simulink model "balancingController_QP_oneFoot"  (R2014b)
settings: Solver=FixedStepDiscrete  StartTime=0.0  StopTime=simulationTime  FixedStep=Ts  RelTol=1e-3
InitFcn:
  | initBalancingController_QP_oneFoot;
undefined symbols (not defined in the file): Aineq_F, amplitudesOscillationsOnOneFoot, bineq_F, directionOfOscillation, frequenciesOscillationsOnOneFoot, gainMomentum, gainsDCOM, gainsICOM, gainsPCOM, impedances, impedencesSat, increasingRatesImp, init_params_QP, localName, number_of_feet_on_ground, referenceParams, robotName, Ts
libraries: WBCLibrary x27
settings Model: Creator=daniele  LastModifiedBy=pucci
settings OptimizationCC: ExpressionDepthLimit=2147483647
settings DebuggingCC: UnderspecifiedInitializationDetection=Classic  MergeDetectMultiDrivingBlocksExec=none  FcnCallInpInsideContextMsg=EnableAllAsWarning  StateNameClashWarn=warning
settings SFSimCC: SimParseCustomCode=off
settings GRTTargetCC: CombineOutputUpdateFcns=off  GRTInterface=on

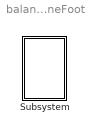
== system balancingController_QP_oneFoot ==
  Subsystem : Subsystem  mask{robotName=robotName, Ts=Ts, localName=localName}
      mask prompts: robotName "robot name"; localName "module name"

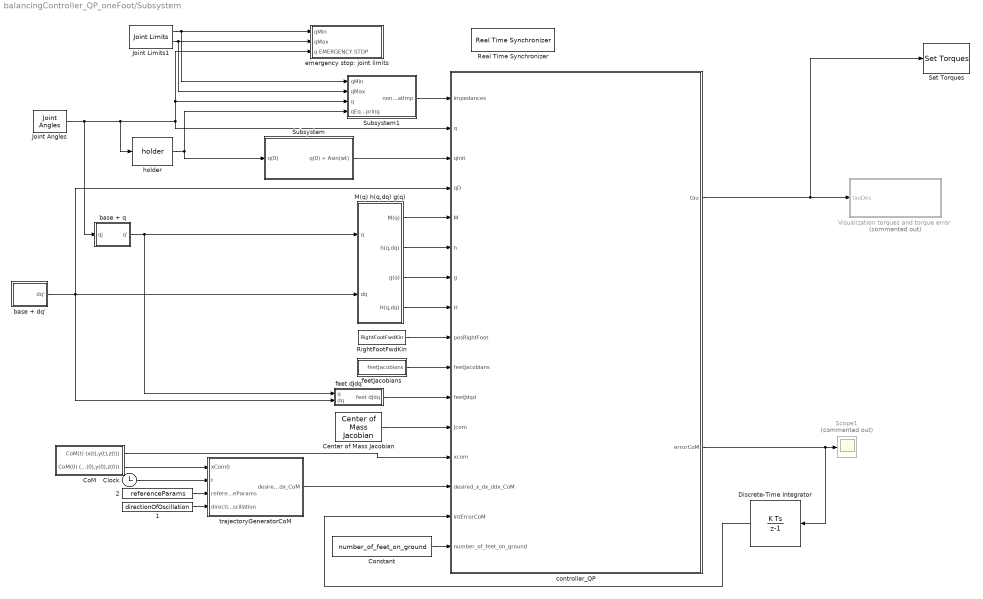
== system balancingController_QP_oneFoot/Subsystem ==
  " 1" : Constant  Value=directionOfOscillation
  " 2" : Constant  Value=referenceParams
  Center of Mass Jacobian : WBCLibrary/wholeBodyModel/Jacobians/Center of Mass Jacobian  robotName=robotName  localName=localName
  Clock : Clock
  "CoM " : Subsystem
  Constant : Constant  Value=number_of_feet_on_ground
  Discrete-Time Integrator : DiscreteIntegrator  InitialCondition=[0 0 0]  SampleTime=Ts
  Joint Angles : WBCLibrary/wholeBodyStates/Joint Angles  robotName=robotName  localName=localName
  Joint Limits1 : WBCLibrary/wholeBodyModel/Joint Limits  robotName=robotName  localName=localName
  M(q) h(q,dq) g(q) : Subsystem
  Real Time Synchronizer : WBCLibrary/Utilities/Real Time Synchronizer  Priority=-10  threadPeriod=Ts
  RightFootFwdKin : WBCLibrary/wholeBodyModel/Forward Kinematics/RightFootFwdKin  robotName=robotName  localName=localName
  Scope1 : Scope  Commented=on
      settings: SaveName=ScopeData6
  Set Torques : WBCLibrary/wholeBodyActuators/Set Torques  val=6  robotName=robotName  localName=localName
  Subsystem : Subsystem
  Subsystem1 : Subsystem
  Visualization torques and torque error : Subsystem  Commented=on
  base + dq' : Subsystem
  base + q : Subsystem
  controller_QP : Subsystem
  emergency stop: joint limits : Subsystem
  feet dJdq : Subsystem
  feetJacobians : Subsystem
  "holder " : WBCLibrary/Utilities/holder 
  trajectoryGeneratorCoM : MATLAB Function  TreatAsAtomicUnit=on
  wires:
  trajectoryGeneratorCoM/1(desired_x_dx_ddx_CoM) -> controller_QP/14(desired_x_dx_ddx_CoM)
  "CoM "/2(CoM(0) (x(0),y(0),z(0))) -> trajectoryGeneratorCoM/1(xCom0)
  RightFootFwdKin/1 -> controller_QP/9(posRightFoot)
  Discrete-Time Integrator/1 -> controller_QP/15(intErrorCoM)
  base + q/1(q') -> M(q) h(q,dq) g(q)/1(q), feet dJdq/1(q)
  M(q) h(q,dq) g(q)/3(g(q)) -> controller_QP/7(g)
  M(q) h(q,dq) g(q)/4(H(q,dq)) -> controller_QP/8(H)
  Center of Mass Jacobian/1 -> controller_QP/12(Jcom)
  feetJacobians/1(feetJacobians) -> controller_QP/10(feetJacobians)
  feet dJdq/1(feet dJdq) -> controller_QP/11(feetJdqd)
  "holder "/1 -> Subsystem1/4(qEquSpring), Subsystem/1(q(0))
  "CoM "/1(CoM(t) (x(t),y(t),z(t))) -> controller_QP/13(xcom)
  base + dq'/1(dq') -> controller_QP/4(qD), M(q) h(q,dq) g(q)/2(dq), feet dJdq/2(dq)
  M(q) h(q,dq) g(q)/1(M(q)) -> controller_QP/5(M)
  M(q) h(q,dq) g(q)/2(h(q,dq)) -> controller_QP/6(h)
  controller_QP/2(errorCoM) -> Scope1/1, Discrete-Time Integrator/1
  Constant/1 -> controller_QP/16(number_of_feet_on_ground)
  controller_QP/1(tau) -> Visualization torques and torque error/1(tauDes), Set Torques/1
  " 2"/1 -> trajectoryGeneratorCoM/3(referenceParams)
  Clock/1 -> trajectoryGeneratorCoM/2(t)
  Subsystem1/1(nonLinSatImp) -> controller_QP/1(impedances)
  Joint Limits1/1 -> emergency stop: joint limits/1(qMin), Subsystem1/1(qMin)
  Joint Limits1/2 -> emergency stop: joint limits/2(qMax), Subsystem1/2(qMax)
  Joint Angles/1 -> base + q/1(qj), "holder "/1, emergency stop: joint limits/3(q EMERGENCY STOP), Subsystem1/3(q), controller_QP/2(q)
  " 1"/1 -> trajectoryGeneratorCoM/4(directionOfOscillation)
  Subsystem/1(q(0) + Asin(wt)) -> controller_QP/3(qInit)

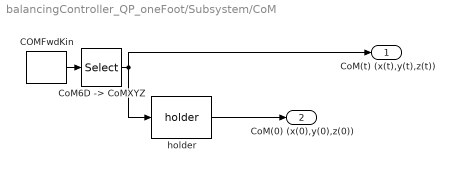
== system balancingController_QP_oneFoot/Subsystem/CoM  ==
  "COMFwdKin " : WBCLibrary/wholeBodyModel/Forward Kinematics/COMFwdKin   robotName=robotName  localName=localName
  "CoM6D -> CoMXYZ" : Selector  InputPortWidth=7  Indices=[1 2 3]
  "holder " : WBCLibrary/Utilities/holder 
  CoM(t) (x(t),y(t),z(t)) : Outport
  CoM(0) (x(0),y(0),z(0)) : Outport  Port=2
  wires:
  "COMFwdKin "/1 -> "CoM6D -> CoMXYZ"/1
  "CoM6D -> CoMXYZ"/1 -> "holder "/1, CoM(t) (x(t),y(t),z(t))/1
  "holder "/1 -> CoM(0) (x(0),y(0),z(0))/1

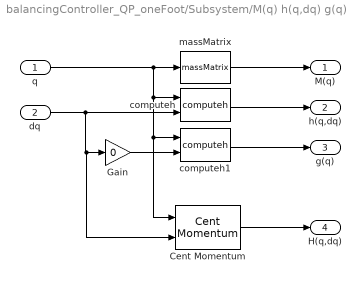
== system balancingController_QP_oneFoot/Subsystem/M(q) h(q,dq) g(q) ==
  q : Inport
  dq : Inport  Port=2
  Cent Momentum : WBCLibrary/wholeBodyModel/Dynamics/Cent Momentum  robotName=robotName  localName=localName
  Gain : Gain  Gain=0
  computeh : WBCLibrary/wholeBodyModel/Dynamics/computeh  val=7  robotname=robotName  localname=localName
  computeh1 : WBCLibrary/wholeBodyModel/Dynamics/computeh  val=7  robotname=robotName  localname=localName
  massMatrix : WBCLibrary/wholeBodyModel/Dynamics/massMatrix  val=8  robotname=robotName  localname=localName
  M(q) : Outport
  h(q,dq) : Outport  Port=2
  g(q) : Outport  Port=3
  H(q,dq) : Outport  Port=4
  wires:
  Gain/1 -> computeh1/2
  computeh1/1 -> g(q)/1
  computeh/1 -> h(q,dq)/1
  massMatrix/1 -> M(q)/1
  q/1 -> Cent Momentum/1, computeh1/1, computeh/1, massMatrix/1
  dq/1 -> Cent Momentum/2, Gain/1, computeh/2
  Cent Momentum/1 -> H(q,dq)/1

== system balancingController_QP_oneFoot/Subsystem/Subsystem ==
  q(0) : Inport
  Sine Wave : Sin  Amplitude=amplitudesOscillationsOnOneFoot*pi/180  Frequency=frequenciesOscillationsOnOneFoot*2*pi  SampleTime=0
  Sum1 : Sum  Inputs=++|
  q(0) + Asin(wt) : Outport
  wires:
  q(0)/1 -> Sum1/2
  Sine Wave/1 -> Sum1/1
  Sum1/1 -> q(0) + Asin(wt)/1

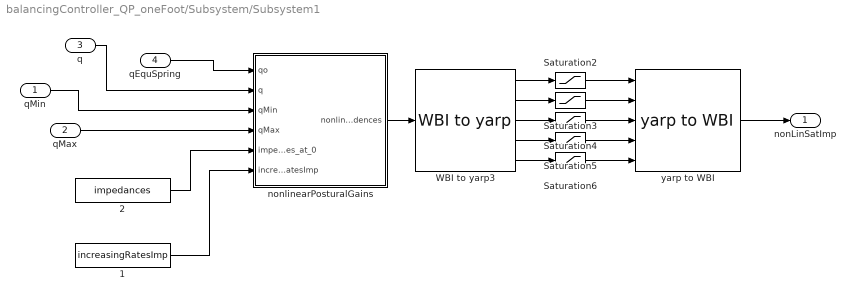
== system balancingController_QP_oneFoot/Subsystem/Subsystem1 ==
  qMin : Inport
  qMax : Inport  Port=2
  q : Inport  Port=3
  qEquSpring : Inport  Port=4
  " 1" : Constant  Value=increasingRatesImp
  " 2" : Constant  Value=impedances
  Saturation2 : Saturate  UpperLimit=impedencesSat(1)  LowerLimit=0  SampleTime=Ts
  Saturation3 : Saturate  UpperLimit=impedencesSat(2)  LowerLimit=0  SampleTime=Ts
  Saturation4 : Saturate  UpperLimit=impedencesSat(2)  LowerLimit=0  SampleTime=Ts
  Saturation5 : Saturate  UpperLimit=impedencesSat(3)  LowerLimit=0  SampleTime=Ts
  Saturation6 : Saturate  UpperLimit=impedencesSat(3)  LowerLimit=0  SampleTime=Ts
  WBI to yarp3 : WBCLibrary/Utilities/WBI to yarp
  "nonlinearPosturalGains " : MATLAB Function  TreatAsAtomicUnit=on
  yarp to WBI : WBCLibrary/Utilities/yarp to WBI
  nonLinSatImp : Outport
  wires:
  WBI to yarp3/1 -> Saturation2/1
  WBI to yarp3/2 -> Saturation3/1
  WBI to yarp3/3 -> Saturation4/1
  WBI to yarp3/4 -> Saturation5/1
  WBI to yarp3/5 -> Saturation6/1
  "nonlinearPosturalGains "/1(nonlinearImpedences) -> WBI to yarp3/1
  yarp to WBI/1 -> nonLinSatImp/1
  qMin/1 -> "nonlinearPosturalGains "/3(qMin)
  qMax/1 -> "nonlinearPosturalGains "/4(qMax)
  " 2"/1 -> "nonlinearPosturalGains "/5(impedences_at_0)
  " 1"/1 -> "nonlinearPosturalGains "/6(increasingRatesImp)
  q/1 -> "nonlinearPosturalGains "/2(q)
  Saturation6/1 -> yarp to WBI/5
  Saturation4/1 -> yarp to WBI/3
  Saturation3/1 -> yarp to WBI/2
  Saturation2/1 -> yarp to WBI/1
  qEquSpring/1 -> "nonlinearPosturalGains "/1(qo)
  Saturation5/1 -> yarp to WBI/4

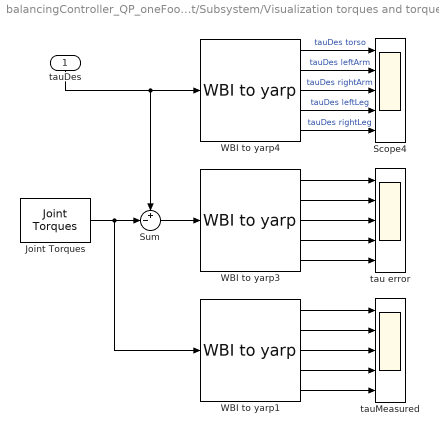
== system balancingController_QP_oneFoot/Subsystem/Visualization torques and torque error ==
  tauDes : Inport
  Joint Torques : WBCLibrary/wholeBodyStates/Joint Torques  robotName=robotName  localName=localName
  Scope4 : Scope  NumInputPorts=5
      settings: ShowLegends=on  TimeRange=132.17  YMin=-30~-4~-5~-40~-5  YMax=10~4~10~40~15  SaveName=ScopeData9
  Sum : Sum  Inputs=+-|
  WBI to yarp1 : WBCLibrary/Utilities/WBI to yarp
  WBI to yarp3 : WBCLibrary/Utilities/WBI to yarp
  WBI to yarp4 : WBCLibrary/Utilities/WBI to yarp
  tau error : Scope  NumInputPorts=5
      settings: YMin=-5~-5~-5~-5~-5  YMax=5~5~5~5~5
  tauMeasured : Scope  NumInputPorts=5
      settings: YMin=-5~-5~-5~-5~-5  YMax=5~5~5~5~5  SaveName=ScopeData7
  wires:
  tauDes/1 -> WBI to yarp4/1, Sum/1
  WBI to yarp4/2 -> Scope4/2  "tauDes leftArm"
  Sum/1 -> WBI to yarp3/1
  Joint Torques/1 -> WBI to yarp1/1, Sum/2
  WBI to yarp4/4 -> Scope4/4  "tauDes leftLeg"
  WBI to yarp4/1 -> Scope4/1  "tauDes torso"
  WBI to yarp4/3 -> Scope4/3  "tauDes rightArm"
  WBI to yarp1/4 -> tauMeasured/4
  WBI to yarp1/2 -> tauMeasured/2
  WBI to yarp1/5 -> tauMeasured/5
  WBI to yarp3/5 -> tau error/5
  WBI to yarp3/3 -> tau error/3
  WBI to yarp1/1 -> tauMeasured/1
  WBI to yarp3/4 -> tau error/4
  WBI to yarp3/2 -> tau error/2
  WBI to yarp4/5 -> Scope4/5  "tauDes rightLeg"
  WBI to yarp3/1 -> tau error/1
  WBI to yarp1/3 -> tauMeasured/3

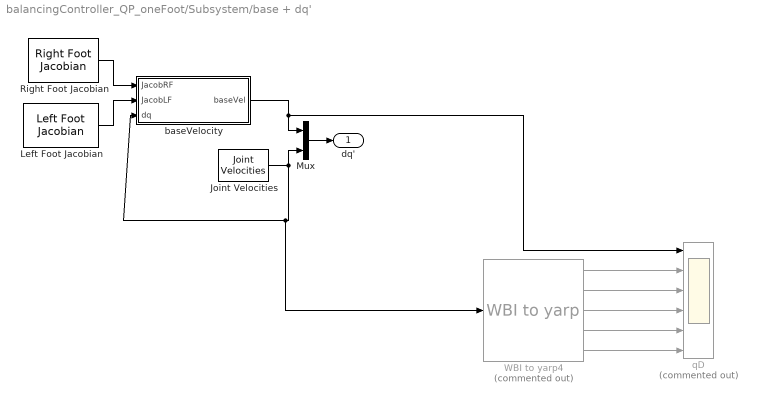
== system balancingController_QP_oneFoot/Subsystem/base + dq' ==
  Joint Velocities : WBCLibrary/wholeBodyStates/Joint Velocities  robotName=robotName  localName=localName
  Left Foot Jacobian : WBCLibrary/wholeBodyModel/Jacobians/Left Foot Jacobian  robotName=robotName  localName=localName
  Mux : Mux  Inputs=2
  Right Foot Jacobian : WBCLibrary/wholeBodyModel/Jacobians/Right Foot Jacobian  robotName=robotName  localName=localName
  WBI to yarp4 : WBCLibrary/Utilities/WBI to yarp  Commented=on
  baseVelocity : Subsystem  AncestorBlock=WBCLibrary/Utilities/baseVelocity  mask(baseVelocity){}
      mask help: This block computes the velocity of the floating base of a bipedal robot
  qD : Scope  Commented=on  NumInputPorts=6
      settings: YMin=-5~-5~-5~-5~-5~-5  YMax=5~5~5~5~5~5  SaveName=ScopeData8
  dq' : Outport
  wires:
  Left Foot Jacobian/1 -> baseVelocity/2(JacobLF)
  Right Foot Jacobian/1 -> baseVelocity/1(JacobRF)
  baseVelocity/1(baseVel) -> qD/1, Mux/1
  Joint Velocities/1 -> WBI to yarp4/1, baseVelocity/3(dq), Mux/2
  Mux/1 -> dq'/1
  WBI to yarp4/1 -> qD/2
  WBI to yarp4/2 -> qD/3
  WBI to yarp4/3 -> qD/4
  WBI to yarp4/4 -> qD/5
  WBI to yarp4/5 -> qD/6

== system balancingController_QP_oneFoot/Subsystem/base + q ==
  qj : Inport
  Constant1 : Constant  Value=zeros(16,1)
  Mux : Mux  Inputs=2
  q' : Outport
  wires:
  Mux/1 -> q'/1
  qj/1 -> Mux/2
  Constant1/1 -> Mux/1

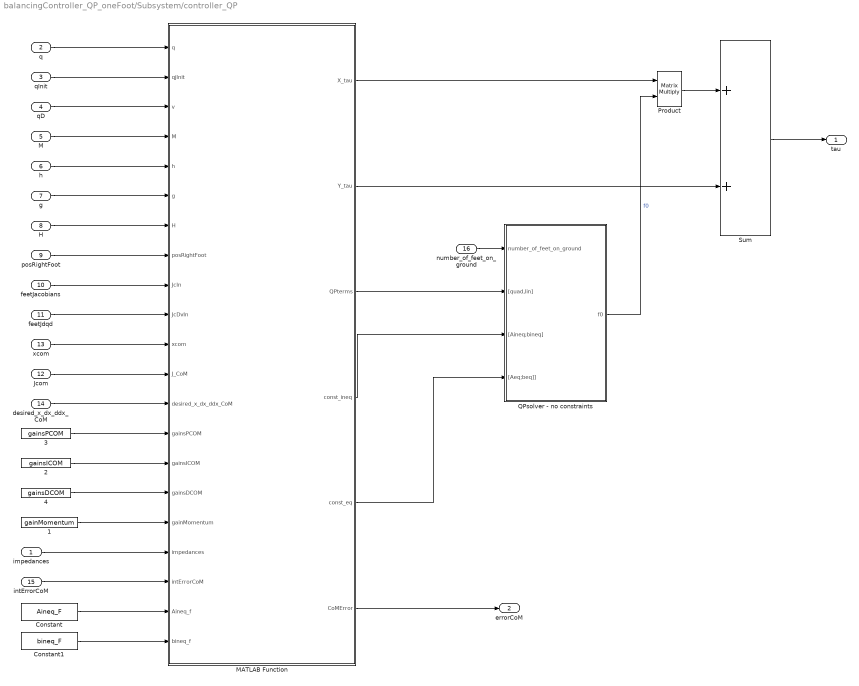
== system balancingController_QP_oneFoot/Subsystem/controller_QP ==
  impedances : Inport
  q : Inport  Port=2
  qInit : Inport  Port=3
  qD : Inport  Port=4
  M : Inport  Port=5
  h : Inport  Port=6
  g : Inport  Port=7
  H : Inport  Port=8
  posRightFoot : Inport  Port=9
  feetJacobians : Inport  Port=10
  feetJdqd : Inport  Port=11
  Jcom : Inport  Port=12
  xcom : Inport  Port=13
  desired_x_dx_ddx_CoM : Inport  Port=14
  intErrorCoM : Inport  Port=15
  number_of_feet_on_ground : Inport  Port=16
  " 1" : Constant  Value=gainMomentum
  " 2" : Constant  Value=gainsICOM
  " 3" : Constant  Value=gainsPCOM
  " 4" : Constant  Value=gainsDCOM
  Constant : Constant  Value=Aineq_F
  Constant1 : Constant  Value=bineq_F
  MATLAB Function : MATLAB Function  TreatAsAtomicUnit=on
  Product : Product  Multiplication=Matrix(*)
  QPsolver - no constraints : Subsystem
  Sum : Sum
  tau : Outport
  errorCoM : Outport  Port=2
  wires:
  q/1 -> MATLAB Function/1(q)
  qInit/1 -> MATLAB Function/2(qjInit)
  qD/1 -> MATLAB Function/3(v)
  M/1 -> MATLAB Function/4(M)
  h/1 -> MATLAB Function/5(h)
  g/1 -> MATLAB Function/6(g)
  H/1 -> MATLAB Function/7(H)
  posRightFoot/1 -> MATLAB Function/8(posRightFoot)
  feetJacobians/1 -> MATLAB Function/9(JcIn)
  feetJdqd/1 -> MATLAB Function/10(JcDvIn)
  xcom/1 -> MATLAB Function/11(xcom)
  Jcom/1 -> MATLAB Function/12(J_CoM)
  desired_x_dx_ddx_CoM/1 -> MATLAB Function/13(desired_x_dx_ddx_CoM)
  impedances/1 -> MATLAB Function/18(impedances)
  intErrorCoM/1 -> MATLAB Function/19(intErrorCoM)
  number_of_feet_on_ground/1 -> QPsolver - no constraints/1(number_of_feet_on_ground)
  MATLAB Function/6(CoMError) -> errorCoM/1
  MATLAB Function/3(QPterms) -> QPsolver - no constraints/2("[quad,lin]")
  MATLAB Function/4(const_ineq) -> QPsolver - no constraints/3("[Aineq;bineq]")
  MATLAB Function/5(const_eq) -> QPsolver - no constraints/4("[Aeq;beq]]")
  QPsolver - no constraints/1(f0) -> Product/2  "f0"
  Sum/1 -> tau/1
  MATLAB Function/1(X_tau) -> Product/1
  Constant/1 -> MATLAB Function/20(Aineq_f)
  Constant1/1 -> MATLAB Function/21(bineq_f)
  " 3"/1 -> MATLAB Function/14(gainsPCOM)
  Product/1 -> Sum/1
  MATLAB Function/2(Y_tau) -> Sum/2
  " 1"/1 -> MATLAB Function/17(gainMomentum)
  " 2"/1 -> MATLAB Function/15(gainsICOM)
  " 4"/1 -> MATLAB Function/16(gainsDCOM)

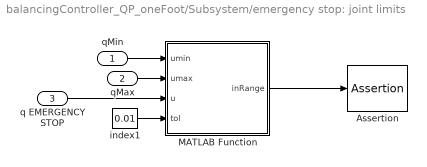
== system balancingController_QP_oneFoot/Subsystem/emergency stop: joint limits ==
  qMin : Inport
  qMax : Inport  Port=2
  q EMERGENCY STOP : Inport  Port=3
  Assertion : Assertion
  MATLAB Function : MATLAB Function  TreatAsAtomicUnit=on
  index1 : Constant  Value=0.01  VectorParams1D=off
  wires:
  qMin/1 -> MATLAB Function/1(umin)
  qMax/1 -> MATLAB Function/2(umax)
  index1/1 -> MATLAB Function/4(tol)
  q EMERGENCY STOP/1 -> MATLAB Function/3(u)
  MATLAB Function/1(inRange) -> Assertion/1

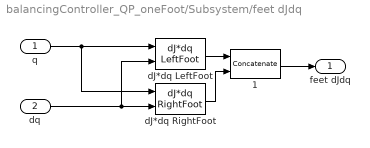
== system balancingController_QP_oneFoot/Subsystem/feet dJdq ==
  q : Inport
  dq : Inport  Port=2
  " 1" : Concatenate  Mode=Multidimensional array
  dJ*dq LeftFoot : WBCLibrary/wholeBodyModel/Dynamics/dJ*dq LeftFoot  val=9  robotName=robotName  localName=localName
  dJ*dq RightFoot : WBCLibrary/wholeBodyModel/Dynamics/dJ*dq RightFoot  val=9  robotName=robotName  localName=localName
  feet dJdq : Outport
  wires:
  dJ*dq LeftFoot/1 -> " 1"/1
  dJ*dq RightFoot/1 -> " 1"/2
  " 1"/1 -> feet dJdq/1
  q/1 -> dJ*dq RightFoot/1, dJ*dq LeftFoot/1
  dq/1 -> dJ*dq LeftFoot/2, dJ*dq RightFoot/2

== system balancingController_QP_oneFoot/Subsystem/feetJacobians ==
  " " : Concatenate  Mode=Multidimensional array
  Left Foot Jacobian : WBCLibrary/wholeBodyModel/Jacobians/Left Foot Jacobian  robotName=robotName  localName=localName
  Right Foot Jacobian : WBCLibrary/wholeBodyModel/Jacobians/Right Foot Jacobian  robotName=robotName  localName=localName
  feetJacobians : Outport
  wires:
  Left Foot Jacobian/1 -> " "/1
  Right Foot Jacobian/1 -> " "/2
  " "/1 -> feetJacobians/1

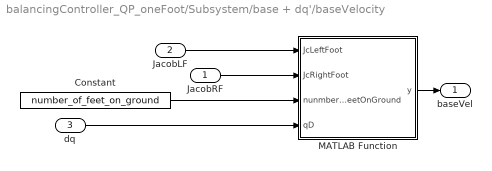
== system balancingController_QP_oneFoot/Subsystem/base + dq'/baseVelocity ==
  JacobRF : Inport
  JacobLF : Inport  Port=2
  dq : Inport  Port=3
  Constant : Constant  Value=number_of_feet_on_ground
  MATLAB Function : MATLAB Function  TreatAsAtomicUnit=on
  baseVel : Outport
  wires:
  JacobLF/1 -> MATLAB Function/1(JcLeftFoot)
  JacobRF/1 -> MATLAB Function/2(JcRightFoot)
  MATLAB Function/1(y) -> baseVel/1
  dq/1 -> MATLAB Function/4(qD)
  Constant/1 -> MATLAB Function/3(nunmberOfFeetOnGround)

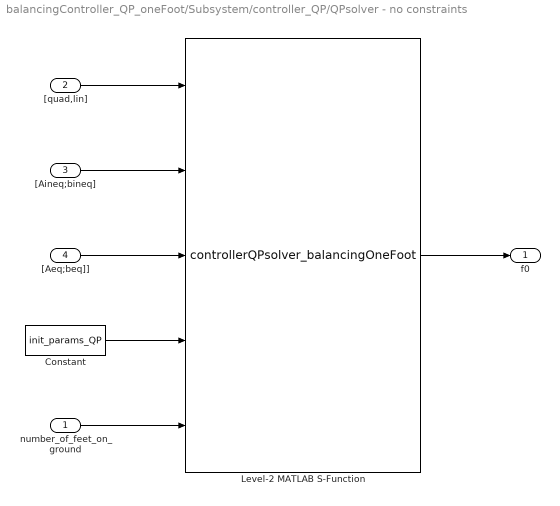
== system balancingController_QP_oneFoot/Subsystem/controller_QP/QPsolver - no constraints ==
  number_of_feet_on_ground : Inport
  "[quad,lin]" : Inport  Port=2
  "[Aineq;bineq]" : Inport  Port=3
  "[Aeq;beq]]" : Inport  Port=4
  Constant : Constant  Value=init_params_QP
  Level-2 MATLAB S-Function : M-S-Function  FunctionName=controllerQPsolver_balancingOneFoot
  f0 : Outport
  wires:
  "[quad,lin]"/1 -> Level-2 MATLAB S-Function/1
  "[Aineq;bineq]"/1 -> Level-2 MATLAB S-Function/2
  "[Aeq;beq]]"/1 -> Level-2 MATLAB S-Function/3
  Constant/1 -> Level-2 MATLAB S-Function/4
  Level-2 MATLAB S-Function/1 -> f0/1
  number_of_feet_on_ground/1 -> Level-2 MATLAB S-Function/5

== matlab function balancingController_QP_oneFoot/Subsystem/trajectoryGeneratorCoM ==
  data: desired_x_dx_ddx_CoM output; xCom0 input; t input; referenceParams input; directionOfOscillation input
function desired_x_dx_ddx_CoM = fcn(xCom0,t,referenceParams,directionOfOscillation)
%#codegen


A = referenceParams(1);
f = referenceParams(2);

xcomDes    = xCom0 + A*sin(2*pi*f*t)*directionOfOscillation;
% xcomDes(1) =  xcomDes(1) + 0.01;
xDcomDes   =         A*2*pi*f*cos(2*pi*f*t)*directionOfOscillation;
xDDcomDes  =        -A*(2*pi*f)^2*sin(2*pi*f*t)*directionOfOscillation;

desired_x_dx_ddx_CoM = [xcomDes,xDcomDes,xDDcomDes];

== matlab function balancingController_QP_oneFoot/Subsystem/base + dq'/baseVelocity/MATLAB Function ==
  data: JcLeftFoot input; JcRightFoot input; nunmberOfFeetOnGround input; y output; qD input
function y = fcn(JcLeftFoot,JcRightFoot,nunmberOfFeetOnGround,qD)
%#codegen
if nunmberOfFeetOnGround == 2
    Jc = [JcLeftFoot;JcRightFoot];
else
    Jc = JcLeftFoot;
end
y = -pinv(Jc(:,1:6))*Jc(:,7:end)*qD;

== matlab function balancingController_QP_oneFoot/Subsystem/controller_QP/MATLAB Function ==
  data: q input; X_tau output; Y_tau output; QPterms output; const_ineq output; const_eq output; qjInit input; v input; M input; h input; g input; H input; posRightFoot input; JcIn input; JcDvIn input; xcom input; J_CoM input; desired_x_dx_ddx_CoM input; gainsPCOM input; gainsICOM input; gainsDCOM input; gainMomentum input; impedances input; intErrorCoM input; CoMError output; Aineq_f input; bineq_f input
function [X_tau,Y_tau,QPterms,const_ineq,const_eq,CoMError]  =  fcnQP_part1(q,qjInit,v, M, h, g, H, posRightFoot, JcIn, JcDvIn, xcom,J_CoM, desired_x_dx_ddx_CoM, gainsPCOM,gainsICOM,gainsDCOM,gainMomentum, impedances, intErrorCoM,Aineq_f,bineq_f)
   
number_of_feet_on_ground =1;
n_dof           = 23;
PINV_TOL        = 1e-5;
regularPinv     = 1e-2;
gravAcc         = 9.81;
m               = M(1,1);
Mb              = M(1:6,1:6);
Mbj             = M(1:6,7:end);
Mj              = M(7:end,7:end);

St              = [  zeros(6,n_dof);
                   eye(n_dof,n_dof)];
grav            = [ zeros(2,1);
                   -m*gravAcc;
                    zeros(3,1)];
pos_rightFoot   = posRightFoot(1:3);

switch number_of_feet_on_ground
    case 1 % on left foot
        A  = [ eye(3),   zeros(3);
             -Sf(xcom),  eye(3)];
         Jc = JcIn(1:6,:);
         JcDv = JcDvIn(1:6);
         pinvA         = inv(A);
    case 2 % on both feet
        A  = [ eye(3),   zeros(3),eye(3), zeros(3);
             -Sf(xcom),  eye(3), Sf(Pr), eye(3) ];
         Jc = JcIn;
         JcDv = JcDvIn;
         pinvA         = pinv(        A, PINV_TOL);
    otherwise
        disp('Choose number of constraints properly (1 or 2)');
        return
end        



JcMinv          = Jc/M;
JcMinvSt        = JcMinv*St;
JcMinvJct       = JcMinv*transpose(Jc);
xDcom           = J_CoM(1:3,:)*v;
qD              = v(7:end);
xDDcomStar      = desired_x_dx_ddx_CoM(:,3) - gainsPCOM*(xcom - desired_x_dx_ddx_CoM(:,1)) - gainsICOM*intErrorCoM - gainsDCOM*(xDcom - desired_x_dx_ddx_CoM(:,2));
Pr              = pos_rightFoot - xcom; % Application point of the contact force on the right foot w.r.t. CoM



% PInv_JcMinvStNoDamp = pinv(JcMinvSt, PINV_TOL);


PInv_JcMinvSt = JcMinvSt'/(JcMinvSt*JcMinvSt' + regularPinv*eye(size(JcMinvSt,1)));


HDotDes  = [ m*xDDcomStar ;
            -gainMomentum*H(4:end)]; 
         
%% QP FOR TORQUE MINIMIZATION BASED ON arbitrary vector F0
% Maux = [     eye(3)     zeros(3,22)
%           zeros(22,3)      inv(Mj(4:end,4:end))];
%define tau_0 (the arbitrary vector)
N0_tau        = eye(n_dof) - PInv_JcMinvSt*JcMinvSt;

mult_f_tau0   =  Mbj'/Mb*transpose(Jc(:,1:6))-transpose(Jc(:,7:end)); % multiplier of f in tau0
n_tau0        =  g(7:end) - impedances.*(q-qjInit)   - Mbj'/Mb*h(1:6) ; % additional terms in tau0 - Mj*(kPandD_Postural(1,:)'.*(q-qjInit) + kPandD_Postural(2,:)'.*qD) 
%

mult_f_tau    = PInv_JcMinvSt*(-JcMinvJct)+N0_tau*mult_f_tau0;
n_tau         = PInv_JcMinvSt*(JcMinv*h-JcDv)+N0_tau*n_tau0;

PInv_JcMinvStJcMinv_h_JcDv = PInv_JcMinvSt*(JcMinv*h-JcDv);
N0_taun_tau0  = N0_tau*n_tau0;

% f desired is given as:
% f*   = pinvA*(HDotDes - grav)  + (I-pinvA*A) * f0
% f*   =           c_f           +     N0_f    * f0
N0_f          = eye(6*number_of_feet_on_ground,6*number_of_feet_on_ground)-pinvA*A;
c_f           = pinvA*(HDotDes - grav);

% tau is given as:
% tau = (mult_f_tau*N0_f)* f0 + (n_tau+mult_f_tau*c_f)
% tau =        X_tau     * f0 +                   Y_tau

X_tau         = mult_f_tau*N0_f;

Y_tau         = n_tau + mult_f_tau*c_f;
quadraticTerm = 2*(transpose(X_tau)*X_tau)+eye(6*number_of_feet_on_ground)*1e-8;
linearTerm    = transpose(2*X_tau'*Y_tau);

% rewrite constraints in terms of f0
Aineq = Aineq_f*N0_f;
bineq = bineq_f-Aineq_f*c_f;

Aeq = zeros(1,6*number_of_feet_on_ground);
beq = zeros(1,1);

QPterms     = reshape([quadraticTerm;linearTerm],1,[]);
const_ineq  = reshape([Aineq,bineq],1,[]);
const_eq    = reshape([Aeq,beq],1,[]);
CoMError    = xcom - desired_x_dx_ddx_CoM(:,1);

== matlab function balancingController_QP_oneFoot/Subsystem/emergency stop: joint limits/MATLAB Function ==
  data: umin input; umax input; u input; inRange output; tol input
function inRange = checkRange(umin, umax, u, tol)
%#codegen

res = u < umin + tol | u > umax - tol;
res = sum(res);
if res==0
    inRange = 1;
else
    inRange = 0;
    u < umin + tol | u > umax - tol
end

== matlab function balancingController_QP_oneFoot/Subsystem/Subsystem1/nonlinearPosturalGains  ==
  data: qo input; nonlinearImpedences output; q input; qMin input; qMax input; impedences_at_0 input; increasingRatesImp input
function nonlinearImpedences = fcn(qo,q,qMin,qMax,impedences_at_0,increasingRatesImp)
    %#codegen

    tp =  pi./(2*(qMax-qo));
    tn = -pi./(2*(qMin-qo));

    qTilde = q - qo;
            
    nonlinearImpedences = impedences_at_0' + (increasingRatesImp.*tan((tp.*stepFcn(qTilde) + tn.*stepFcn(-qTilde)).*qTilde).^2)' ;
end

function y = stepFcn(x) 
   %#codegen
   y = x > 0; 
end
